simulink model "first_order_system_RL"  (R2020a)
settings: Solver=VariableStepAuto  StartTime=0.0  StopTime=10.0  RelTol=1e-3
InitFcn:
  | V=220;
  | L=100;
  | R=22;
libraries: powerlib x5
settings Model: Creator=User  LastModifiedBy=User

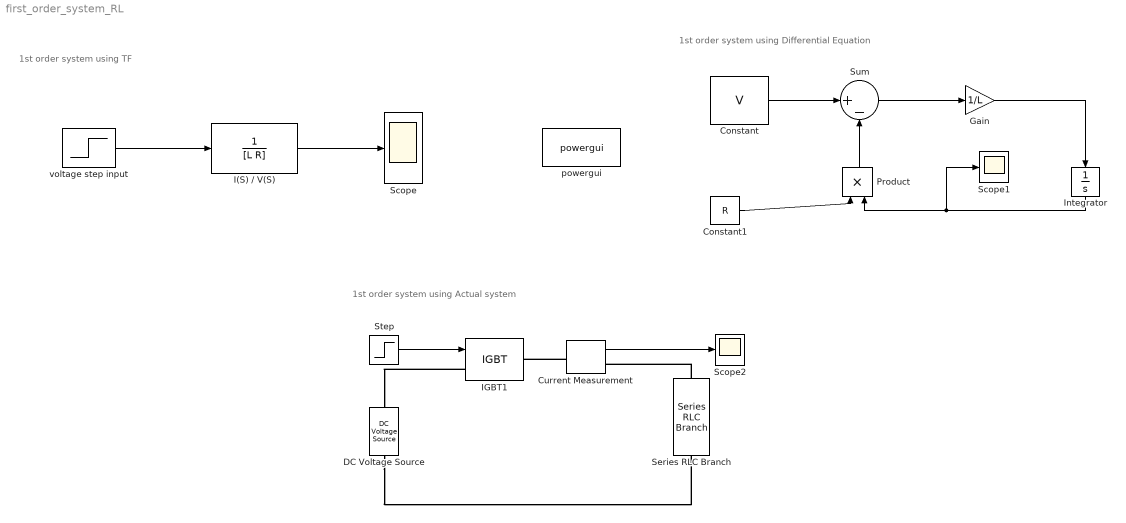
== system first_order_system_RL ==
  note: 1st order system using Actual system
  note: 1st order system using Differential Equation
  note: 1st order system using TF
  Constant : Constant  Value=V
  Constant1 : Constant  Value=R
  Current Measurement : powerlib/Measurements/Current Measurement  PhasorSimulation=off  OutputType=Complex  PSBequivalent=0
  DC Voltage Source : powerlib/Electrical Sources/DC Voltage Source  Amplitude=V  Measurements=None
  Gain : Gain  Gain=1/L
  I(S) / V(S) : TransferFcn  Denominator=[L R]
  IGBT1 : powerlib/Power Electronics/IGBT  Ron=0.001  Lon=0  Vf=1  Tf=1e-6  Tt=2e-6  IC=0  Rs=1e5  Cs=inf  Measurements=off
  Integrator : Integrator
  Product : Product
  Scope : Scope
  Scope1 : Scope
  Scope2 : Scope
  Series RLC Branch : powerlib/Elements/Series RLC Branch  LConnTagsString=__new0  RConnTagsString=__new0  BranchType=RL  Resistance=R  Inductance=L  SetiL0=off  InitialCurrent=0  Capacitance=1e-6  Setx0=off  InitialVoltage=0  Measurements=None
  Step : Step  SampleTime=0
  Sum : Sum  Inputs=|+-
  powergui : powerlib/powergui  Priority=1  SimulationMode=Continuous  SampleTime=50e-6  frequency=60  Iterations=50  frequencyindice=0  Pbase=100e6  ErrMax=1e-4  UnitsV=kV  UnitsW=MW  buscounter=0  FunctionMessages=off  echomessages=off  EnableUseOfTLC=off  CurrentSourceSwitches=off  DisableSnubberDevices=on  DisableRonSwitches=on  DisableVfSwitches=on  DisplayEquations=off  AutomaticDiscreteSolvers=off  SolverType=Tustin/Backward Euler (TBE)  Interpol=off  ExternalGateDelay=off  methode=off  Ts=100  x0status=blocks  SPID=on  SwTol=0  HookPort=off  NonlinearTolerance=1e-4  nMaxIteration=100  ContinueOnMaxIteration=off  RestoreLinks=warning  ResistiveCurrentMeasurement=off  Frange=[0:2:500]  Ylog=off  Xlog=on  ShowGrid=off  save=off  variable=ZData  structure=0  ZoomFFT=off  StartTime=0.0  cycles=1  DisplayStyle=1  fundamental=60  FreqAxis=off  MaxFrequency=1000  frequencyindicesteady=1  RmsSteady=1  display=off
  voltage step input : Step  After=V  SampleTime=0
  wires:
  voltage step input/1 -> I(S) / V(S)/1
  I(S) / V(S)/1 -> Scope/1
  Constant/1 -> Sum/1
  Product/1 -> Sum/2
  Constant1/1 -> Product/1
  Sum/1 -> Gain/1
  Gain/1 -> Integrator/1
  Integrator/1 -> Scope1/1, Product/2
  Current Measurement/1 -> Scope2/1
  Step/1 -> IGBT1/1
  connections:
  IGBT1/LConn1 -- DC Voltage Source/RConn1
  DC Voltage Source/LConn1 -- Series RLC Branch/LConn1
  Current Measurement/LConn1 -- IGBT1/RConn1
  Series RLC Branch/RConn1 -- Current Measurement/RConn1
